simulink model "sm_pid"  (R2025b)
settings: Solver=VariableStepAuto  StartTime=0.0  StopTime=40  MaxStep=0.01  RelTol=1e-3
values from neighbouring files (symbols this model uses):
  kd = gaina(3)    [findkp_ki_kd.m]
  ki = gaina(2)    [findkp_ki_kd.m]
  kp = gaina(1)    [findkp_ki_kd.m]
libraries: cstblocks x1
settings Model: Creator=AIZAZ BADRU  LastModifiedBy=AIZAZ BADRU

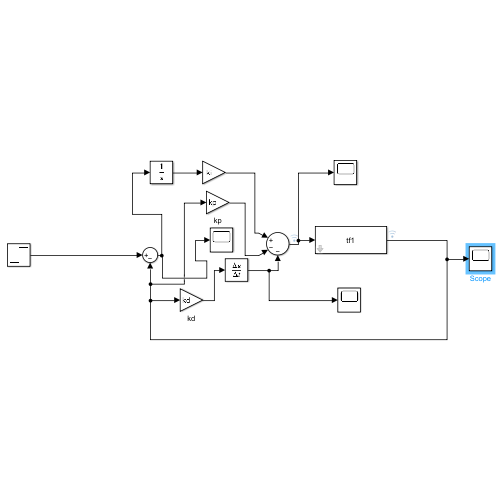
[thumbnail: Simulink's stored preview of the top-level diagram]
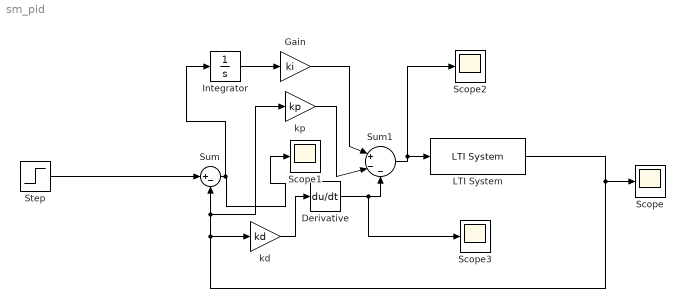
== system sm_pid ==
  Derivative : Derivative
  Gain : Gain  Gain=ki
  Integrator : Integrator
  LTI System : cstblocks/LTI System  sys=tf1  IC=[]  PadeOrder=0
  Scope{,1..3} (4 alike) : Scope
      Scope settings: ActiveDisplayYMinimum=-26.887737672512102  ActiveDisplayYMaximum=186.35524268489169
      Scope1 settings: ActiveDisplayYMinimum=-1  ActiveDisplayYMaximum=1
      Scope2 settings: ActiveDisplayYMinimum=-759.79556056727631  ActiveDisplayYMaximum=878.45210725198183  DataLoggingVariableName=ScopeData2
      Scope3 settings: ActiveDisplayYMinimum=-1  ActiveDisplayYMaximum=1  DataLoggingVariableName=ScopeData3
  Step : Step  Time=0  After=100  SampleTime=0
  Sum : Sum  Inputs=|+-
  Sum1 : Sum  Inputs=|+--
  kd : Gain  Gain=kd
  kp : Gain  Gain=kp
  wires:
  Sum1/1 -> Scope2/1, LTI System/1
  Sum/1 -> Integrator/1, Scope1/1
  Integrator/1 -> Gain/1
  Gain/1 -> Sum1/1
  kp/1 -> Sum1/2
  kd/1 -> Derivative/1
  Derivative/1 -> Scope3/1, Sum1/3
  Step/1 -> Sum/1
  LTI System/1 -> kd/1, kp/1, Sum/2, Scope/1
